simulink model "Motor_Test_Boat"  (Simulink 7.3)
settings: Solver=FixedStepDiscrete  StartTime=0.0  StopTime=inf  FixedStep=1  RelTol=1e-3
undefined symbols (not defined in the file): RPM1, RPM2
settings Model: Creator=gclayton  LastModifiedBy=wildcat  SimulationMode=external
settings RTWCC: SystemTargetFile=rlnx.tlc  GenCodeOnly=on  TemplateMakefile=rlnx_ubuntu.tmf  Description=Linux Real-Time Target  ProcessScript=rlnx_make_rtw_hook
settings CodeAppCC: GenerateComments=off  SimulinkBlockComments=off
settings STFCustomTargetCC: ModelReferenceCompliant=off  MatFileLogging=on  SystemTargetFile=rlnx.tlc
settings GRTTargetCC: ModelReferenceCompliant=off  ParMdlRefBuildCompliant=off  CompOptLevelCompliant=off  ExtMode=on  ExtModeMexArgs='10.0.0.2'
settings CustomProperty: DataType=string  Value=/matlab_includes/libfreenect/build/lib/libfreenect.so -lm -ldl
settings EnumStrPairs: String=PC

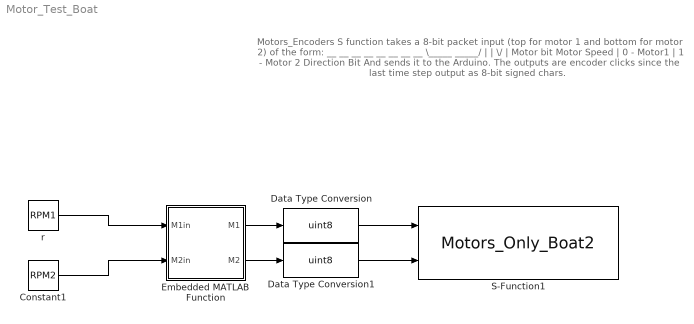
== system Motor_Test_Boat ==
  note: Motors_Encoders S function takes a 8-bit packet input
      | (top for motor 1 and bottom for motor 2) of the form:
      |
      |          __ __ __ __ __ __ __ __
      |         \_____   _____/   |    |
      |                               \/              |  Motor bit
      |                          Motor Speed    |   0 - Motor1
      |                                                    |   1 - Motor 2
      |                                Direction Bit
      |
      | And sends it to the Arduino.  The outputs are encoder clicks
      | since the last time step output as 8-bit signed chars.
  Constant1 : Constant  Value=RPM2  OutDataType=fixdt(1, 16)  OutScaling=2^0
  Data Type Conversion : DataTypeConversion  OutDataTypeMode=uint8  OutDataType=fixdt(1, 16)  OutScaling=2^0  OutDataTypeStr=uint8
  Data Type Conversion1 : DataTypeConversion  OutDataTypeMode=uint8  OutDataType=fixdt(1, 16)  OutScaling=2^0  OutDataTypeStr=uint8
  Embedded MATLAB Function : Stateflow chart
  S-Function1 : S-Function  FunctionName=Motors_Only_Boat2  EnableBusSupport=off
  r : Constant  Value=RPM1  OutDataType=fixdt(1, 16)  OutScaling=2^0
  wires:
  Embedded MATLAB Function/1(M1) -> Data Type Conversion/1
  Embedded MATLAB Function/2(M2) -> Data Type Conversion1/1
  Data Type Conversion/1 -> S-Function1/1
  Data Type Conversion1/1 -> S-Function1/2
  r/1 -> Embedded MATLAB Function/1(M1in)
  Constant1/1 -> Embedded MATLAB Function/2(M2in)

== matlab function Embedded MATLAB Function ==
  data: M1in input double; M1 output double; M2in input double; M2 output double
function [M1, M2] = MotorPackets(M1in, M2in)
%#eml

M1 = 0;
M2 = 1;

if M1in <= 0
    M1 = M1+2;
end

if M2in <= 0
    M2 = M2+2;
end

M1 = M1 + round(abs(M1in)/15)*4;
M2 = M2 + round(abs(M2in)/15)*4;
